simulink model "OpenLoop"  (R2015b)
settings: Solver=ode1  StartTime=0.0  StopTime=200  FixedStep=0.002  RelTol=1e-3
values from neighbouring files (symbols this model uses):
  A = [0,1,0,0,0,0;0,0,0,0,0,0;0,0,0,1,0,0;0,0,0,0,0,0;0,0,0,0,0,1;0,0,0,0,0,0]    [ProportionalController.m]    (also in SecondOrderResponse.m = (log(PO/100))^2)
  B = [0,0,0;(1/Ix),0,0;0,0,0;0,(1/Iy),0;0,0,0;0,0,(1/Iz)]    [ProportionalController.m]
  C = [1,0,0,0,0,0;0,1,0,0,0,0;0,0,1,0,0,0]    [ProportionalController.m]
  D = [0,0,0;0,0,0;0,0,0]    [ProportionalController.m]
  K_AMP = 3    [ProportionalController.m]
  VMAX_DAC = 10    [ProportionalController.m]
  wcf = 2 * pi * 20    (= 125.663706144)    [ProportionalController.m]
  zetaf = 0.6    [ProportionalController.m]
libraries: simulink_extras x1
settings Model: ExtModeTrigDuration=10000  Creator=rmh66  LastModifiedBy=rmh66
settings SolverCC: PositivePriorityOrder=on
settings RTWCC: SystemTargetFile=quarc_win64.tlc  TemplateMakefile=quarc_default_tmf  Description=QUARC Win64 Target
settings STFCustomTargetCC: GeneratePreprocessorConditionals=Use local settings  CPPClassGenCompliant=off
settings GRTTargetCC: ParMdlRefBuildCompliant=off  CompOptLevelCompliant=off  CombineOutputUpdateFcns=off  MatFileLogging=off  CPPClassGenCompliant=off  GRTInterface=on  UseToolchainInfoCompliant=off  ExtMode=on  ExtModeMexFile=quarc_comm

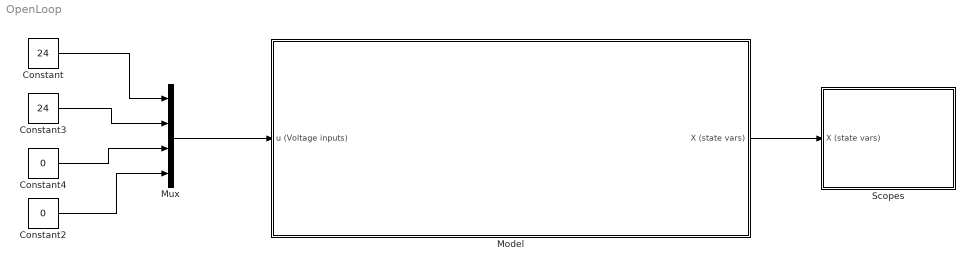
== system OpenLoop ==
  Constant : Constant  Value=24
  Constant2 : Constant  Value=0
  Constant3 : Constant  Value=24
  Constant4 : Constant  Value=0
  "Model " : Subsystem
  Mux : Mux
  Scopes : Subsystem
  wires:
  "Model "/1(X (state vars)) -> Scopes/1(X (state vars))
  Mux/1 -> "Model "/1(u (Voltage inputs))
  Constant/1 -> Mux/1
  Constant2/1 -> Mux/4
  Constant3/1 -> Mux/2
  Constant4/1 -> Mux/3

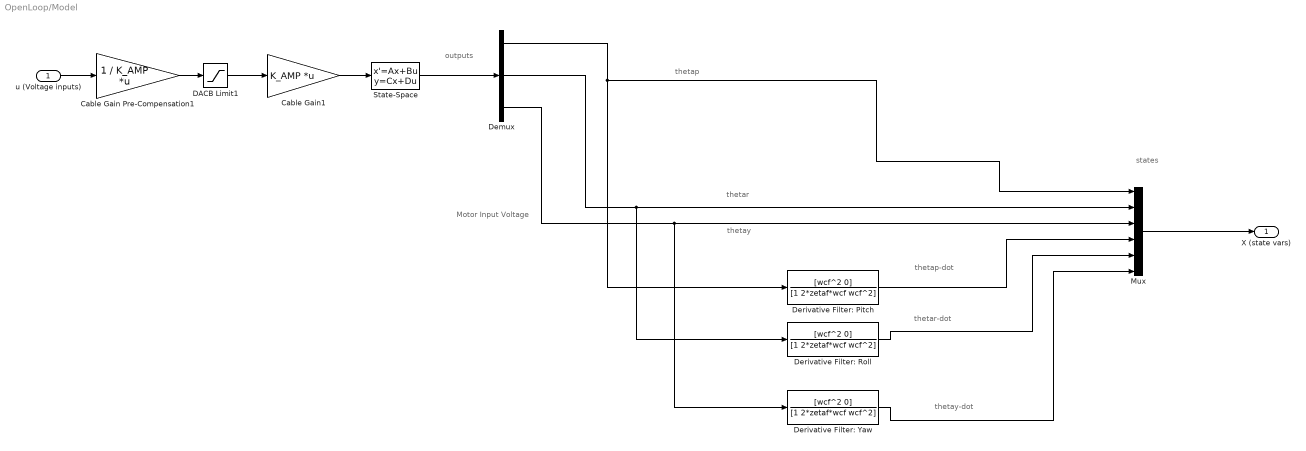
== system OpenLoop/Model  ==
  note: states
  note: thetap
  note: thetar
  note: thetay
  note: outputs
  note: thetap-dot
  note: thetar-dot
  note: thetay-dot
  note: Motor Input Voltage
  u (Voltage inputs) : Inport
  Cable Gain Pre-Compensation1 : Gain  Gain=1 / K_AMP  Multiplication=Matrix(K*u)  SaturateOnIntegerOverflow=on  OutDataTypeStr=Inherit: Same as input  ParamDataTypeStr=Inherit: Same as input
  Cable Gain1 : Gain  Gain=K_AMP  Multiplication=Matrix(K*u)  SaturateOnIntegerOverflow=on  OutDataTypeStr=Inherit: Same as input  ParamDataTypeStr=Inherit: Same as input
  DACB Limit1 : Saturate  UpperLimit=VMAX_DAC  LowerLimit=-VMAX_DAC
  Demux : Demux  Outputs=3
  Derivative Filter: Pitch : TransferFcn  Numerator=[wcf^2 0]  Denominator=[1 2*zetaf*wcf wcf^2]
  Derivative Filter: Roll : TransferFcn  Numerator=[wcf^2 0]  Denominator=[1 2*zetaf*wcf wcf^2]
  Derivative Filter: Yaw : TransferFcn  Numerator=[wcf^2 0]  Denominator=[1 2*zetaf*wcf wcf^2]
  Mux : Mux  Inputs=6
  State-Space : StateSpace  A=A  B=B  C=C  D=D  X0=0
  X (state vars) : Outport
  wires:
  State-Space/1 -> Demux/1
  Demux/1 -> Derivative Filter: Pitch/1, Mux/1
  Demux/2 -> Derivative Filter: Roll/1, Mux/2
  Demux/3 -> Derivative Filter: Yaw/1, Mux/3
  Derivative Filter: Pitch/1 -> Mux/4
  Derivative Filter: Roll/1 -> Mux/5
  Derivative Filter: Yaw/1 -> Mux/6
  Mux/1 -> X (state vars)/1
  DACB Limit1/1 -> Cable Gain1/1
  Cable Gain Pre-Compensation1/1 -> DACB Limit1/1
  u (Voltage inputs)/1 -> Cable Gain Pre-Compensation1/1
  Cable Gain1/1 -> State-Space/1

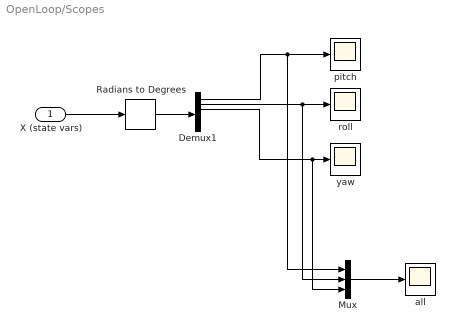
== system OpenLoop/Scopes ==
  X (state vars) : Inport
  Demux1 : Demux  Outputs=6
  Mux : Mux  Inputs=3
  Radians to Degrees : simulink_extras/Transformations/Radians to Degrees
  all : Scope
  pitch : Scope
  roll : Scope
  yaw : Scope
  wires:
  X (state vars)/1 -> Radians to Degrees/1
  Radians to Degrees/1 -> Demux1/1
  Demux1/1 -> Mux/1, pitch/1
  Demux1/2 -> Mux/2, roll/1
  Demux1/3 -> Mux/3, yaw/1
  Mux/1 -> all/1
